simulink model "satellite_adcs_model"  (R2014b)
settings: Solver=ode3  StartTime=0.0  StopTime=tdur  FixedStep=dt  RelTol=1e-3
values from neighbouring files (symbols this model uses):
  CTRL_DT_MODE = 3    [satellite_adcs_run.m]
  CTRL_PT1_MODE = 5    [satellite_adcs_run.m]
  CTRL_PT2_MODE = 5    [satellite_adcs_run.m]
  CTRL_SWITCH1 = 1    [satellite_adcs_run.m]
  CTRL_SWITCH2 = P/2    [satellite_adcs_run.m]
  dt = CONST.dt    [extended_kalman_filter.m]    (also in filter_kalman_extended.m; filter_kalman_sequential.m; filter_kalman_unscented.m; satellite_adcs_run.m = 1)
  dt_gyro = 0.1    [satellite_adcs_run.m]
  dt_mg = dt    (= 1)    [satellite_adcs_run.m]
  dt_ss = dt    (= 1)    [satellite_adcs_run.m]
  dt_st = dt    (= 1)    [satellite_adcs_run.m]
  dt_ts = dt    (= 1)    [satellite_adcs_run.m]
  GYRO_Bias = [0.5;0.2;-0.3]*pi/180    [satellite_adcs_run.m]
  q_B_I_0 = qinvert(q_I_B_0,'xyzw')    [satellite_adcs_run.m]
  R_G_B = dcm(2,pi/2)    [satellite_adcs_run.m]
  R_S1_B = dcm(SSaxis(1),SSangles(1))    [satellite_adcs_run.m]
  R_S2_B = dcm(SSaxis(2),SSangles(2))    [satellite_adcs_run.m]
  R_S3_B = dcm(SSaxis(3),SSangles(3))    [satellite_adcs_run.m]
  R_S4_B = dcm(SSaxis(4),SSangles(4))    [satellite_adcs_run.m]
  sigMag = 1.25e-7    (= 1.25e-07)    [satellite_adcs_run.m]
  sigSS = 0.01*pi/180    (= 0.000174532925199)    [satellite_adcs_run.m]
  Taero_toggle = 0    [satellite_adcs_run.m]
  Tcontrol_toggle = 1    [satellite_adcs_run.m]
  temp_coeff = [0.01; 0.02; 0.005]*pi/180    [satellite_adcs_run.m]
  temp_ref = 20    [satellite_adcs_run.m]
  Tgg_toggle = 0    [satellite_adcs_run.m]
  Tsolar_toggle = 0    [satellite_adcs_run.m]
  Ug = dcm(3,GYRO_Mis(3))*dcm(2,GYRO_Mis(2))*dcm(1,GYRO_Mis(1))    [satellite_adcs_run.m]
  Umg = eye(3) + Gmg    [satellite_adcs_run.m]    (also in sensor_mag.m = CONST.Umg)
  update_st1 = 2    [satellite_adcs_run.m]
  update_st2 = 2    [satellite_adcs_run.m]
  Var_ARW = N_ARW^2    (= 2.56183250041e-09)    [satellite_adcs_run.m]
  Var_RRW = K_RRW^2/3    (= 4.06156559716e-12)    [satellite_adcs_run.m]
  varTemp = sigTemp^2    (= 4e-06)    [satellite_adcs_run.m]
  VarW = N_W^2    (= 3.04617419787e-22)    [satellite_adcs_run.m]
  w_B_BI_0 = w_B_BO_0 + w_B_OI_0    [satellite_adcs_run.m]
  wdot_B_BI_tgt = [0;0;0]    [satellite_adcs_run.m]
undefined symbols (not defined in the file or in its folder): magnitude, R_0, V_0, varST_x, varST_y, varST_z
libraries: simulink x6
(part 2 of 2)

== system satellite_adcs_model/Sensors/Sun Sensor/Sun Sensor 4 ==
  S_B_hat : Inport
  Compare To Constant1 : simulink/Logic and Bit Operations/Compare To Constant  relop=<=  const=3.0  OutDataTypeStr=boolean
  Demux2 : Demux  Outputs=3
  Mux1 : Mux  Inputs=3
  Product : Product
  R_S4_B*(u) : Gain  Gain=R_S4_B  Multiplication=Matrix(K*u)
  SS Noise : RandomNumber  Variance=(sigSS*pi/180)^2  SampleTime=dt_ss
  Sum : Sum  Inputs=++|
  S_S4_m : Outport
  S_S4 : Outport  Port=2
  wires:
  Product/1 -> S_S4_m/1
  R_S4_B*(u)/1 -> S_S4/1, Demux2/1
  Demux2/1 -> Mux1/1
  Demux2/2 -> Mux1/2
  Demux2/3 -> Compare To Constant1/1, Mux1/3
  Compare To Constant1/1 -> Product/2
  S_B_hat/1 -> R_S4_B*(u)/1
  Sum/1 -> Product/1
  SS Noise/1 -> Sum/1
  Mux1/1 -> Sum/2
